simulink model "Module4_No2"  (R2021b)
settings: Solver=FixedStepAuto  StartTime=0.0  StopTime=5.0  RelTol=1e-3
libraries: simulink x4
settings Model: Creator=Lenovo  LastModifiedBy=Lenovo

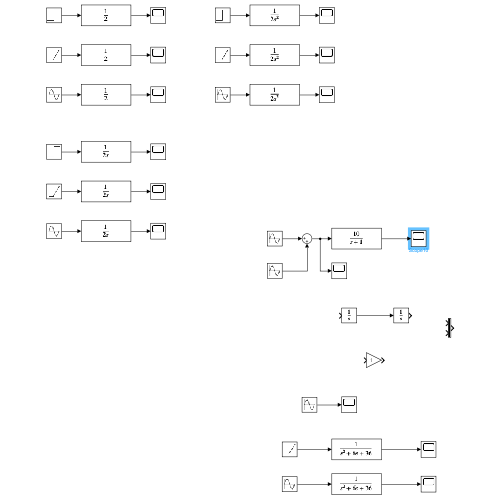
[thumbnail: Simulink's stored preview of the top-level diagram]
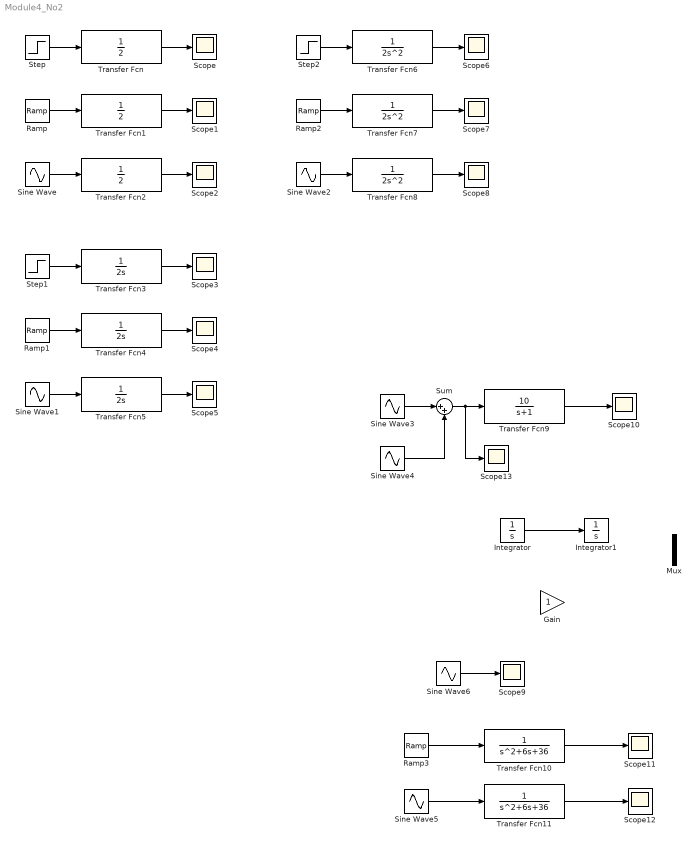
== system Module4_No2 ==
  Gain : Gain
  Integrator : Integrator
  Integrator1 : Integrator
  Mux : Mux  Inputs=2
  Ramp : simulink/Sources/Ramp  slope=1  start=0  InitialOutput=1
  Ramp1 : simulink/Sources/Ramp  slope=1  start=0  InitialOutput=1
  Ramp2 : simulink/Sources/Ramp  slope=1  start=0  InitialOutput=1
  Ramp3 : simulink/Sources/Ramp  slope=2  start=0  InitialOutput=1
  Scope{,1..13} (14 alike) : Scope
  Sine Wave : Sin  Frequency=2*pi  SampleTime=0
  Sine Wave1 : Sin  Frequency=2*pi  SampleTime=0
  Sine Wave2 : Sin  Frequency=2*pi  SampleTime=0
  Sine Wave3 : Sin  Frequency=80*pi  SampleTime=0
  Sine Wave4 : Sin  Frequency=1.5*pi  SampleTime=0
  Sine Wave5 : Sin  Frequency=pi  SampleTime=0
  Sine Wave6 : Sin  Frequency=4*pi  SampleTime=0
  Step : Step  Time=0  SampleTime=0
  Step1 : Step  Time=0  SampleTime=0
  Step2 : Step  Time=0  SampleTime=0
  Sum : Sum  Inputs=|++
  Transfer Fcn : TransferFcn  Denominator=[0 0 2]
  Transfer Fcn1 : TransferFcn  Denominator=[0 0 2]
  Transfer Fcn10 : TransferFcn  Denominator=[1 6 36]
  Transfer Fcn11 : TransferFcn  Denominator=[1 6 36]
  Transfer Fcn2 : TransferFcn  Denominator=[0 0 2]
  Transfer Fcn3 : TransferFcn  Denominator=[0 2 0]
  Transfer Fcn4 : TransferFcn  Denominator=[0 2 0]
  Transfer Fcn5 : TransferFcn  Denominator=[0 2 0]
  Transfer Fcn6 : TransferFcn  Denominator=[2 0 0]
  Transfer Fcn7 : TransferFcn  Denominator=[2 0 0]
  Transfer Fcn8 : TransferFcn  Denominator=[2 0 0]
  Transfer Fcn9 : TransferFcn  Numerator=[10]  Denominator=[0 1 1]
  wires:
  Step/1 -> Transfer Fcn/1
  Transfer Fcn/1 -> Scope/1
  Ramp/1 -> Transfer Fcn1/1
  Transfer Fcn1/1 -> Scope1/1
  Sine Wave/1 -> Transfer Fcn2/1
  Transfer Fcn2/1 -> Scope2/1
  Step1/1 -> Transfer Fcn3/1
  Transfer Fcn3/1 -> Scope3/1
  Ramp1/1 -> Transfer Fcn4/1
  Transfer Fcn4/1 -> Scope4/1
  Transfer Fcn5/1 -> Scope5/1
  Sine Wave1/1 -> Transfer Fcn5/1
  Transfer Fcn6/1 -> Scope6/1
  Transfer Fcn7/1 -> Scope7/1
  Ramp2/1 -> Transfer Fcn7/1
  Transfer Fcn8/1 -> Scope8/1
  Sine Wave2/1 -> Transfer Fcn8/1
  Step2/1 -> Transfer Fcn6/1
  Integrator/1 -> Integrator1/1
  Transfer Fcn9/1 -> Scope10/1
  Sum/1 -> Scope13/1, Transfer Fcn9/1
  Sine Wave3/1 -> Sum/1
  Sine Wave4/1 -> Sum/2
  Ramp3/1 -> Transfer Fcn10/1
  Transfer Fcn10/1 -> Scope11/1
  Transfer Fcn11/1 -> Scope12/1
  Sine Wave5/1 -> Transfer Fcn11/1
  Sine Wave6/1 -> Scope9/1
